simulink model "sphere_portal_mech"  (R2017a)
settings: Solver=FixedStepAuto  StartTime=0.0  StopTime=100  FixedStep=0.001  RelTol=1e-2  EnableMultiTasking=on
undefined symbols (not defined in the file): m, rad, s
libraries: mblibv1 x42, simulink x3, instrumentlib x1
settings Model: SimulationMode=accelerator  Creator=ivanp7  LastModifiedBy=ivanp7
settings OptimizationCC: LifeSpan=inf
settings DebuggingCC: AlgebraicLoopMsg=none  SFUnexpectedBacktrackingDiag=warning  SFNoUnconditionalDefaultTransitionDiag=warning  SFExecutionAtInitializationDiag=none
settings GRTTargetCC: TargetLangStandard=C89/C90 (ANSI)  GeneratePreprocessorConditionals=Disable all
settings ConfigComp: CovMetricSettings=dw  CovHtmlReporting=on  CovSaveCumulativeToWorkspaceVar=on  CovSaveSingleToWorkspaceVar=on  CovExternalEMLEnable=off
settings SimMechanicsCC: LastVizWinPosition=[1141 536 560 420]  CamPosition=[4.37083;-0.373326;26.621;]  CamTarget=[4.37083;-0.373326;0;]  CamUpVector=[0;1;0;]  CamHeight=73.1719  VisBackgroundColor=[0.9;0.9;0.95;]  DefaultBodyColor=[1;0;0;]

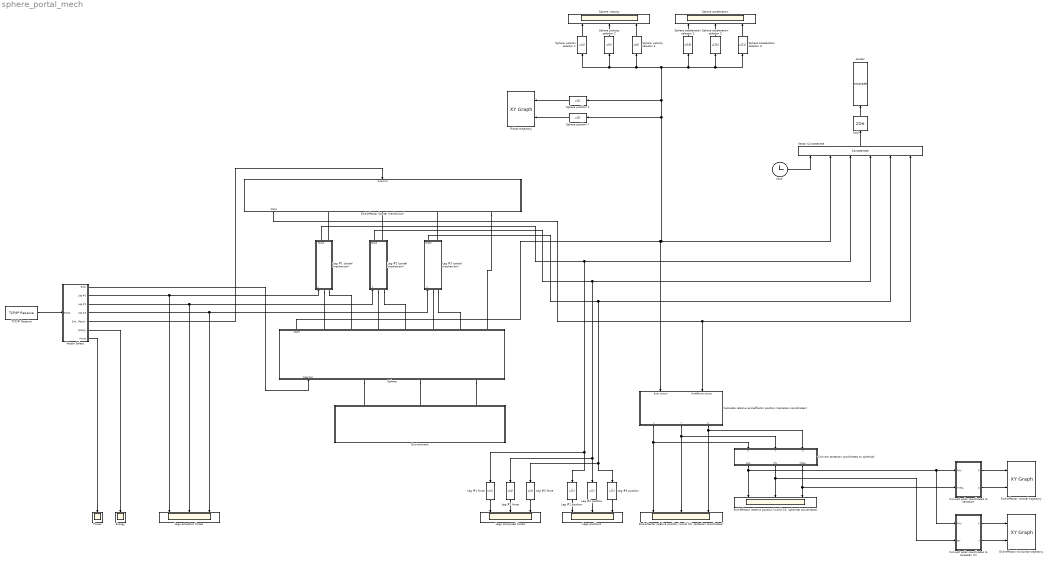
== system sphere_portal_mech ==
  Calculate relative end-effector position (cartesian coordinates) : Subsystem
  Convert cartesian coordinates to spherical : Subsystem
  Convert polar coordinates to cartesian : Subsystem
  Convert polar coordinates to cartesian (2) : Subsystem
  End-effector (portal mechanism) : Subsystem  mask{endeffector_radius=0.2, endeffector_mass=10, endeffector_inertia_coef=2/5}
      mask prompts: endeffector_radius "End-effector radius, m"; endeffector_mass "End-effector mass, kg"; endeffector_inertia_coef "End-effector inertia coefficient"
      mask init:
      | endeffector = endeffector_radius * ...
      |     [[-1; 0; 0], ...
      |      [0; -1; 0], ...
      |      [0; 0; -1], ...
      |      [1; 0; 0], ...
      |      [0; 1; 0], ...
      |      [0; 0; 1]];
  End-effector horizontal trajectory : simulink/Sinks/XY Graph  xmin=-1  xmax=1  ymin=-1  ymax=1  st=-1
  "End-effector relative position (world CS, cartesian coordinates)" : Scope  NumInputPorts=3
  "End-effector relative position (world CS, spherical coordinates)" : Scope  NumInputPorts=3
  End-effector vertical trajectory : simulink/Sinks/XY Graph  xmin=0  xmax=1  ymin=-1  ymax=1  st=-1
  Energy : Scope
  Environment : Subsystem  mask{sphere_radius=1, initial_velocity_x=0, initial_velocity_y=0}
      mask prompts: sphere_radius "Sphere radius, m"; initial_velocity_x "Initial velocity (x-axis), m/s"; initial_velocity_y "Initial velocity (y-axis), m/s"
  Leg #1 force : Fcn  Expr=u(4)
  Leg #1 position : Fcn  Expr=u(1)
  Leg #1 (portal mechanism) : Subsystem  mask{leg_mass=0.1, sphere_radius=1, p_axis=[1 0 0], transient_time=0.001}
      mask prompts: leg_mass "Leg mass, kg"; sphere_radius "Sphere radius, m"; p_axis "Prismatic joint axis"; transient_time "Derivative transient time"
      mask init:
      | p_axis = p_axis / sqrt(sum(p_axis.^2));
      | 
      | v = rand(1, 3);
      | inplane_axis1 = cross(v, p_axis);
      | inplane_axis1 = inplane_axis1 / sqrt(sum(inplane_axis1.^2));
      | inplane_axis2 = cross(inplane_axis1, p_axis);
  Leg #2 force : Fcn  Expr=u(4)
  Leg #2 position : Fcn  Expr=u(1)
  Leg #2 (portal mechanism) : Subsystem  mask{leg_mass=0.1, sphere_radius=1, p_axis=[0 1 0], transient_time=0.001}
      mask prompts: leg_mass "Leg mass, kg"; sphere_radius "Sphere radius, m"; p_axis "Prismatic joint axis"; transient_time "Derivative transient time"
      mask init:
      | p_axis = p_axis / sqrt(sum(p_axis.^2));
      | 
      | v = rand(1, 3);
      | inplane_axis1 = cross(v, p_axis);
      | inplane_axis1 = inplane_axis1 / sqrt(sum(inplane_axis1.^2));
      | inplane_axis2 = cross(inplane_axis1, p_axis);
  Leg #3 force : Fcn  Expr=u(4)
  Leg #3 position : Fcn  Expr=u(1)
  Leg #3 (portal mechanism) : Subsystem  mask{leg_mass=0.1, sphere_radius=1, p_axis=[0 0 1], transient_time=0.001}
      mask prompts: leg_mass "Leg mass, kg"; sphere_radius "Sphere radius, m"; p_axis "Prismatic joint axis"; transient_time "Derivative transient time"
      mask init:
      | p_axis = p_axis / sqrt(sum(p_axis.^2));
      | 
      | v = rand(1, 3);
      | inplane_axis1 = cross(v, p_axis);
      | inplane_axis1 = inplane_axis1 / sqrt(sum(inplane_axis1.^2));
      | inplane_axis2 = cross(inplane_axis1, p_axis);
  Legs actuators forces : Scope  NumInputPorts=3
  Legs computed forces : Scope  NumInputPorts=3
  Legs positions : Scope  NumInputPorts=3
  Power : Scope
  Robot trajectory : simulink/Sinks/XY Graph  xmin=-100  xmax=100  ymin=-100  ymax=100  st=-1
  Sphere : Subsystem  mask{sphere_radius=1, sphere_mass=1, sphere_inertia_coef=2/3}
      mask prompts: sphere_radius "Sphere radius, m"; sphere_mass "Sphere mass, kg"; sphere_inertia_coef "Sphere inertia coefficient, m"
      mask init:
      | cube_side_center = sphere_radius / sqrt(3) * ...
      |     [[-1; 0; 0], ...
      |      [0; -1; 0], ...
      |      [0; 0; -1], ...
      |      [1; 0; 0], ...
      |      [0; 1; 0], ...
      |      [0; 0; 1]];
  Sphere acceleration selector 1 : Fcn  Expr=u(19)
  Sphere acceleration selector 2 : Fcn  Expr=u(20)
  Sphere acceleration selector 3 : Fcn  Expr=u(21)
  Sphere velocity selector 1 : Fcn  Expr=u(4)
  Sphere velocity selector 2 : Fcn  Expr=u(5)
  Sphere velocity selector 3 : Fcn  Expr=u(6)
  Sphere acceleration : Scope  NumInputPorts=3
  Sphere position X : Fcn  Expr=u(1)
  Sphere position Y : Fcn  Expr=u(2)
  Sphere velocity : Scope  NumInputPorts=3
  TCP/IP Receive : instrumentlib/TCP//IP Receive  Priority=1  Host=localhost  Port=61111  DataSize="[1  17]"  EnableBlockingMode=on  Timeout=1  SampleTime=0.001  DataType=double  ByteOrder=LittleEndian
      settings: SourceProductName=Instrument Control Toolbox
  Vector Concatenate : Concatenate  NumInputs=6
  Vector Select : Subsystem
  clock : Clock
      settings: Decimation=1000
  hold : ZeroOrderHold  SampleTime=-1
  sender : M-S-Function  Priority=2  DialogController=instrumentcreatedialog  FunctionName=stcpipsb  Parameters=Host, Port, EnableBlockingMode, Timeout, ByteOrder  DisplayMFileStacktrace=off  mask(TCP/IP Send){Host=localhost, Port=61112, EnableBlockingMode=on, Timeout=1, ByteOrder=LittleEndian}
      mask prompts: Port "Remote Port:"; EnableBlockingMode "Enable blocking mode"; ByteOrder "Byte order:"
      mask help: Send data over TCP/IP network to a specified remote machine.
      mask init:
      | [str port] = instrumentslgate('privateslgetdisplaystring', EnableBlockingMode);
      mask Help: eval('helpview(fullfile(docroot, ''toolbox'', ''instrument'', ''instrument.map''), ''ICT_tcpipsend_Block'')');
      mask TypeOptions ByteOrder: BigEndian | LittleEndian
      mask Display:
      | disp(str);
      | port_label('input',port(1).id,port(1).label);
  wires:
  Leg #1 (portal mechanism)/1(State) -> Leg #1 force/1, Leg #1 position/1, Vector Concatenate/3
  Leg #2 (portal mechanism)/1(State) -> Leg #2 force/1, Leg #2 position/1, Vector Concatenate/4
  Leg #3 (portal mechanism)/1(State) -> Leg #3 force/1, Leg #3 position/1, Vector Concatenate/5
  End-effector (portal mechanism)/1(State) -> Calculate relative end-effector position (cartesian coordinates)/2(Endeffector sensor), Vector Concatenate/6
  Leg #1 position/1 -> Legs positions/1
  Leg #2 position/1 -> Legs positions/2
  Leg #3 position/1 -> Legs positions/3
  Vector Select/4(Leg #3) -> Leg #3 (portal mechanism)/1(Reaction), Legs actuators forces/3
  Vector Select/2(Leg #1) -> Leg #1 (portal mechanism)/1(Reaction), Legs actuators forces/1
  Vector Select/3(Leg #2) -> Leg #2 (portal mechanism)/1(Reaction), Legs actuators forces/2
  Vector Select/5(End effector) -> End-effector (portal mechanism)/1(Reaction)
  Vector Select/1(Body) -> Sphere/1(Reaction)
  Sphere velocity selector 3/1 -> Sphere velocity/3
  Sphere acceleration selector 1/1 -> Sphere acceleration/1
  Sphere acceleration selector 2/1 -> Sphere acceleration/2
  Sphere acceleration selector 3/1 -> Sphere acceleration/3
  Sphere velocity selector 2/1 -> Sphere velocity/2
  Sphere velocity selector 1/1 -> Sphere velocity/1
  Vector Select/6(Energy) -> Energy/1
  Sphere/1(State) -> Vector Concatenate/2, Sphere position X/1, Sphere velocity selector 2/1, Sphere velocity selector 1/1, Sphere velocity selector 3/1, Sphere acceleration selector 1/1, Sphere acceleration selector 2/1, Sphere acceleration selector 3/1, Sphere position Y/1, Calculate relative end-effector position (cartesian coordinates)/1(Body sensor)
  Calculate relative end-effector position (cartesian coordinates)/1(X) -> "End-effector relative position (world CS, cartesian coordinates)"/1, Convert cartesian coordinates to spherical/1(X)
  Calculate relative end-effector position (cartesian coordinates)/2(Y) -> "End-effector relative position (world CS, cartesian coordinates)"/2, Convert cartesian coordinates to spherical/2(Y)
  Calculate relative end-effector position (cartesian coordinates)/3(Z) -> "End-effector relative position (world CS, cartesian coordinates)"/3, Convert cartesian coordinates to spherical/3(Z)
  Convert cartesian coordinates to spherical/1(Rho) -> Convert polar coordinates to cartesian (2)/1(Rho), Convert polar coordinates to cartesian/1(Rho), "End-effector relative position (world CS, spherical coordinates)"/1
  Convert cartesian coordinates to spherical/2(Phi) -> Convert polar coordinates to cartesian (2)/2(Phi), "End-effector relative position (world CS, spherical coordinates)"/2
  Convert cartesian coordinates to spherical/3(Theta) -> Convert polar coordinates to cartesian/2(Theta), "End-effector relative position (world CS, spherical coordinates)"/3
  TCP/IP Receive/1 -> Vector Select/1(Robot)
  hold/1 -> sender/1
  Vector Concatenate/1 -> hold/1
  clock/1 -> Vector Concatenate/1
  Leg #2 force/1 -> Legs computed forces/2
  Leg #1 force/1 -> Legs computed forces/1
  Leg #3 force/1 -> Legs computed forces/3
  Vector Select/7(Power) -> Power/1
  Sphere position X/1 -> Robot trajectory/1
  Sphere position Y/1 -> Robot trajectory/2
  Convert polar coordinates to cartesian/1(R) -> End-effector vertical trajectory/1
  Convert polar coordinates to cartesian/2(Z) -> End-effector vertical trajectory/2
  Convert polar coordinates to cartesian (2)/2(Y) -> End-effector horizontal trajectory/2
  Convert polar coordinates to cartesian (2)/1(X) -> End-effector horizontal trajectory/1
  connections:
  Leg #1 (portal mechanism)/LConn1 -- Sphere/RConn1
  Leg #1 (portal mechanism)/LConn2 -- Sphere/RConn2
  Sphere/LConn1 -- Environment/LConn1
  Sphere/LConn2 -- Environment/LConn2
  Sphere/LConn3 -- Environment/LConn3
  Leg #1 (portal mechanism)/RConn1 -- End-effector (portal mechanism)/RConn1
  End-effector (portal mechanism)/RConn4 -- Sphere/RConn7
  Leg #2 (portal mechanism)/RConn1 -- End-effector (portal mechanism)/RConn2
  Leg #3 (portal mechanism)/RConn1 -- End-effector (portal mechanism)/RConn3
  Leg #2 (portal mechanism)/LConn1 -- Sphere/RConn3
  Leg #2 (portal mechanism)/LConn2 -- Sphere/RConn4
  Leg #3 (portal mechanism)/LConn1 -- Sphere/RConn5
  Leg #3 (portal mechanism)/LConn2 -- Sphere/RConn6

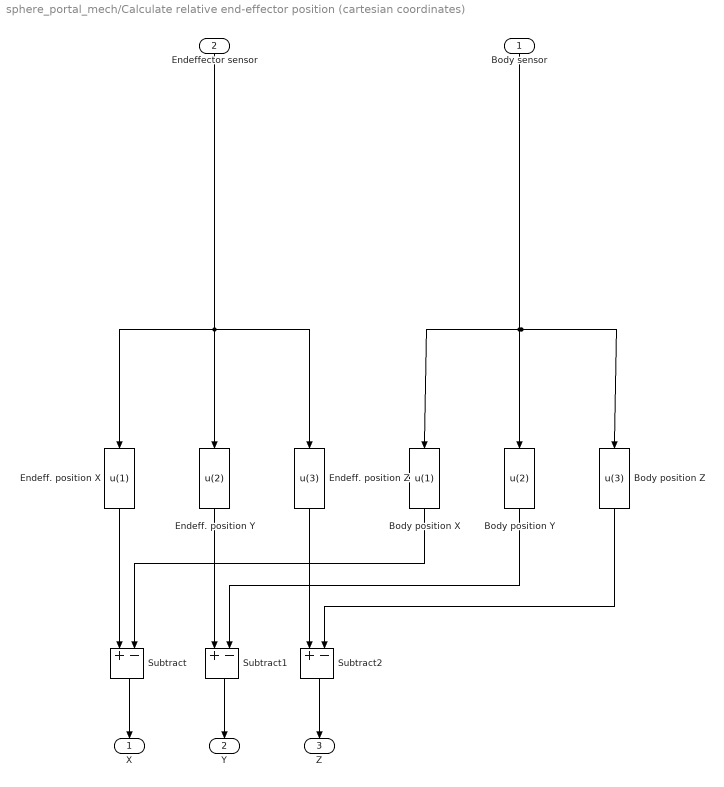
== system sphere_portal_mech/Calculate relative end-effector position (cartesian coordinates) ==
  Body sensor : Inport
  Endeffector sensor : Inport  Port=2
  Body position X : Fcn  Expr=u(1)
  Body position Y : Fcn  Expr=u(2)
  Body position Z : Fcn  Expr=u(3)
  Endeff. position X : Fcn  Expr=u(1)
  Endeff. position Y : Fcn  Expr=u(2)
  Endeff. position Z : Fcn  Expr=u(3)
  Subtract : Sum  Inputs=+-
  Subtract1 : Sum  Inputs=+-
  Subtract2 : Sum  Inputs=+-
  X : Outport
  Y : Outport  Port=2
  Z : Outport  Port=3
  wires:
  Body position X/1 -> Subtract/2
  Body position Z/1 -> Subtract2/2
  Subtract/1 -> X/1
  Subtract1/1 -> Y/1
  Endeff. position X/1 -> Subtract/1
  Endeff. position Y/1 -> Subtract1/1
  Endeff. position Z/1 -> Subtract2/1
  Subtract2/1 -> Z/1
  Body sensor/1 -> Body position Z/1, Body position Y/1, Body position X/1
  Body position Y/1 -> Subtract1/2
  Endeffector sensor/1 -> Endeff. position Z/1, Endeff. position X/1, Endeff. position Y/1

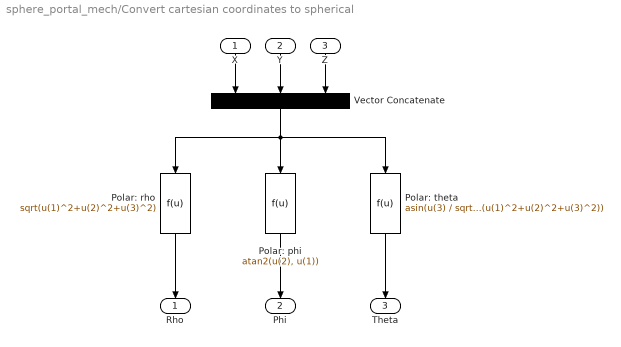
== system sphere_portal_mech/Convert cartesian coordinates to spherical ==
  X : Inport
  Y : Inport  Port=2
  Z : Inport  Port=3
  Polar: phi : Fcn  Expr=atan2(u(2), u(1))
  Polar: rho : Fcn  Expr=sqrt(u(1)^2+u(2)^2+u(3)^2)
  Polar: theta : Fcn  Expr=asin(u(3) / sqrt(u(1)^2+u(2)^2+u(3)^2))
  Vector Concatenate : Concatenate  NumInputs=3
  Rho : Outport
  Phi : Outport  Port=2
  Theta : Outport  Port=3
  wires:
  Polar: rho/1 -> Rho/1
  Polar: phi/1 -> Phi/1
  Polar: theta/1 -> Theta/1
  Y/1 -> Vector Concatenate/2
  Z/1 -> Vector Concatenate/3
  X/1 -> Vector Concatenate/1
  Vector Concatenate/1 -> Polar: theta/1, Polar: rho/1, Polar: phi/1

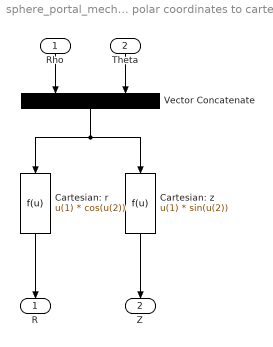
== system sphere_portal_mech/Convert polar coordinates to cartesian ==
  Rho : Inport
  Theta : Inport  Port=2
  Cartesian: r : Fcn  Expr=u(1) * cos(u(2))
  Cartesian: z : Fcn  Expr=u(1) * sin(u(2))
  Vector Concatenate : Concatenate
  R : Outport
  Z : Outport  Port=2
  wires:
  Cartesian: r/1 -> R/1
  Cartesian: z/1 -> Z/1
  Theta/1 -> Vector Concatenate/2
  Rho/1 -> Vector Concatenate/1
  Vector Concatenate/1 -> Cartesian: z/1, Cartesian: r/1

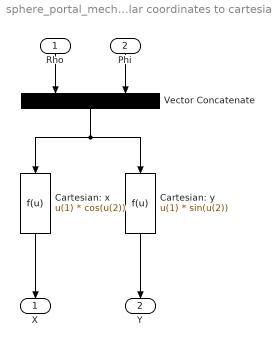
== system sphere_portal_mech/Convert polar coordinates to cartesian (2) ==
  Rho : Inport
  Phi : Inport  Port=2
  Cartesian: x : Fcn  Expr=u(1) * cos(u(2))
  Cartesian: y : Fcn  Expr=u(1) * sin(u(2))
  Vector Concatenate : Concatenate
  X : Outport
  Y : Outport  Port=2
  wires:
  Cartesian: x/1 -> X/1
  Cartesian: y/1 -> Y/1
  Phi/1 -> Vector Concatenate/2
  Rho/1 -> Vector Concatenate/1
  Vector Concatenate/1 -> Cartesian: y/1, Cartesian: x/1

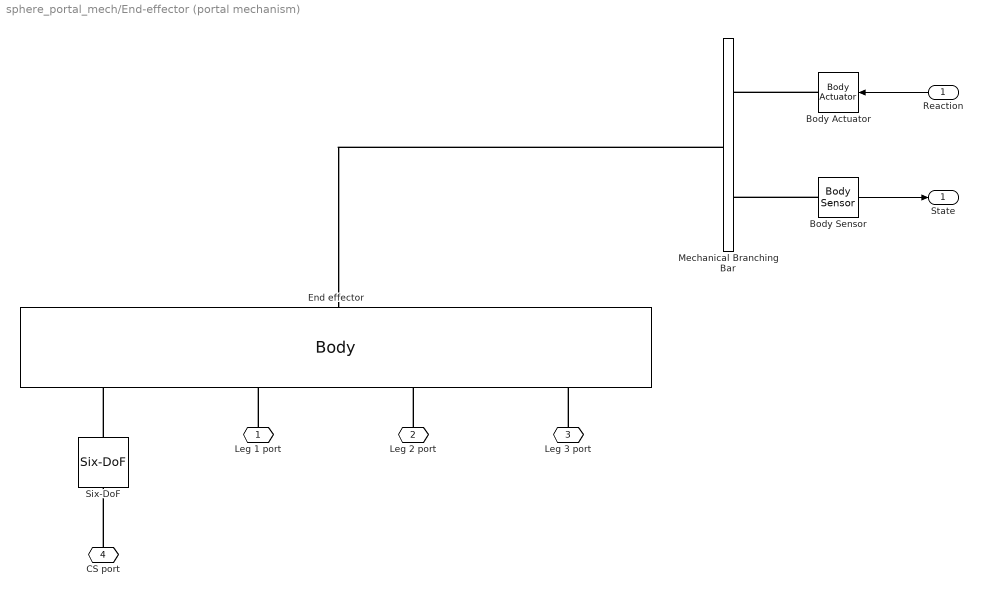
== system sphere_portal_mech/End-effector (portal mechanism) ==
  Reaction : Inport  OutDataTypeStr=double
  Body Actuator : mblibv1/Sensors &  Actuators/Body Actuator  UpdateFromCAD=off  PhysicalDomain=Mechanical  PortType=blob  ActuationStyle=Force  AngleUnits=deg  ArcVelocityUnits=deg/s  ArcAccelerationUnits=deg/s^2  CoordPositionUnits=m  VelocityUnits=m/s  AccelerationUnits=m/s^2  ForceUnits=N  TorqueUnits=N*m  ActiveIO=on  Width=6  DialogClass=MechanicalActuatorBlock  ReferenceFrame=Absolute (World)  Angle=off  CoordPosition=on  Force=on  Torque=on
      settings: SourceProductName=Simscape Multibody  SourceProductBaseCode=MS
  Body Sensor : mblibv1/Sensors &  Actuators/Body Sensor  UpdateFromCAD=off  PhysicalDomain=Mechanical  PortType=blob  Muxed=on  Pose=on  Angle=on  AngleUnits=deg  ArcVelocity=on  ArcVelocityUnits=rad/s  ArcAcceleration=on  ArcAccelerationUnits=rad/s^2  CoordPosition=on  CoordPositionUnits=m  Velocity=on  VelocityUnits=m/s  Acceleration=on  AccelerationUnits=m/s^2  Quaternion=on  QuaternionDT=off  QuaternionDDT=off  QuaternionUnits=off  OutputVector=[1]  ActiveIO=on  Width=24  DialogClass=MechanicalSensorBlock  ReferenceFrame=Absolute (World)
      settings: SourceProductName=Simscape Multibody  SourceProductBaseCode=MS
  End effector : mblibv1/Bodies/Body  LConnTagsString=CS7  RConnTagsString=CG|CS8|CS9|CS10  UpdateFromCAD=off  DialogClass=MechanicalBodyBlock  Mass=endeffector_mass  MassUnits=kg  InertiaUnits=kg*m^2  Inertia=endeffector_inertia_coef*endeffector_mass*endeffector_radius^2*eye(3)  Shape=Cylinder  ShapeDims=[1 1]  ShapeUnits=m  ShapeUse=false  Density=1  DensityUnits=kg/m^3  DensityUse=false  GraphicsMode=CONVHULL  BodyColorSelMode=MACHINE_DEFAULT  BodyColor=[1 0 0]  AttachedToCS=CG  CG=Right$CG$[0;0;0]$Adjoining$Adjoining$m$[0 0 0]$Euler X-Y-Z$deg$Adjoining$true$none  WorkingFrames=Right$CS1$endeffector(:, 1)$CG$CG$m$[0 0 0]$Euler X-Y-Z$deg$CG$false$none#Right$CS2$endeffector(:, 2)$CG$CG$m$[0 0 0]$Euler X-Y-Z$deg$CG$false$none#Right$CS3$endeffector(:, 3)$CG$CG$m$[0 0 0]$Euler X-Y-Z$deg$CG$false$none#Right$CS4$endeffector(:, 4)$CG$CG$m$[0 0 0]$Euler X-Y-Z$deg$CG$false$none#Right$CS5$endeffector(:, 5)$CG$CG$m$[0 0 0]$Euler X-Y-Z$deg$CG$false$none#Right$CS6$endeffector(:, 6)$CG$CG$m$[0 0 0]$Euler X-Y-Z$deg$CG$false$none#Left$CS7$[0;0;0]$CG$CG$m$[0 0 0]$Euler X-Y-Z$deg$CG$true$none#Right$CS8$[0;0;0]$CG$CG$m$[0 0 0]$Euler X-Y-Z$deg$CG$true$none#Right$CS9$[0;0;0]$CG$CG$m$[0 0 0]$Euler X-Y-Z$deg$CG$true$none#Right$CS10$[0;0;0]$CG$CG$m$[0 0 0]$Euler X-Y-Z$deg$CG$true$none  CGPos=[0;0;0]  CGRot=[0 0 0]  CS0Pos=[]  CS0Rot=[]  CS1Pos=endeffector(:, 1)  CS1Rot=[0 0 0]  CS2Pos=endeffector(:, 2)  CS2Rot=[0 0 0]  CS3Pos=endeffector(:, 3)  CS3Rot=[0 0 0]  CS4Pos=endeffector(:, 4)  CS4Rot=[0 0 0]  CS5Pos=endeffector(:, 5)  CS5Rot=[0 0 0]  CS6Pos=endeffector(:, 6)  CS6Rot=[0 0 0]  CS7Pos=[0;0;0]  CS7Rot=[0 0 0]  CS8Pos=[0;0;0]  CS8Rot=[0 0 0]  CS9Pos=[0;0;0]  CS9Rot=[0 0 0]  CS10Pos=[0;0;0]  CS10Rot=[0 0 0]  CS11Pos=[]  CS11Rot=[]  CS12Pos=[]  CS12Rot=[]  CS13Pos=[]  CS13Rot=[]  CS14Pos=[]  CS14Rot=[]  CS15Pos=[]  CS15Rot=[]  CS16Pos=[]  CS16Rot=[]  CS17Pos=[]  CS17Rot=[]  CS18Pos=[]  CS18Rot=[]  CS19Pos=[]  CS19Rot=[]  CS20Pos=[]  CS20Rot=[]
      settings: SourceProductName=Simscape Multibody  SourceProductBaseCode=MS
  Mechanical Branching Bar : mblibv1/Utilities/Mechanical Branching Bar  LConnTagsString=_newl0  RConnTagsString=SA0|SA1  UpdateFromCAD=off  DialogClass=MechanicalBranchingBarBlock  NumSAPorts=2
      settings: SourceProductName=Simscape Multibody  SourceProductBaseCode=MS
  Six-DoF : mblibv1/Joints/Six-DoF  LConnTagsString=__newl0  RConnTagsString=__newr0  UpdateFromCAD=off  NumSAPorts=0  CutJoint=off  MarkAsCut=off  Primitives=prismatic_prismatic  PrimitiveProps=P1$WORLD$[1 0 0]$prismatic#P2$WORLD$[0 1 0]$prismatic#P3$WORLD$[0 0 1]$prismatic#S$WORLD$[0 0 0]$spherical  DialogClass=JointBlock  P1Axis=[1 0 0]  P2Axis=[0 1 0]  P3Axis=[0 0 1]  SAxis=[0 0 0]
      settings: SourceProductName=Simscape Multibody  SourceProductBaseCode=MS
  Leg 1 port : PMIOPort  Port=1  Side=Right
  Leg 2 port : PMIOPort  Port=2  Side=Right
  Leg 3 port : PMIOPort  Port=3  Side=Right
  CS port : PMIOPort  Port=4  Side=Right
  State : Outport  OutDataTypeStr=double
  wires:
  Reaction/1 -> Body Actuator/1
  Body Sensor/1 -> State/1
  connections:
  Mechanical Branching Bar/LConn1 -- End effector/LConn1
  Leg 2 port/RConn1 -- End effector/RConn3
  Leg 3 port/RConn1 -- End effector/RConn4
  Leg 1 port/RConn1 -- End effector/RConn2
  Body Actuator/RConn1 -- Mechanical Branching Bar/RConn1
  Six-DoF/RConn1 -- End effector/RConn1
  Body Sensor/LConn1 -- Mechanical Branching Bar/RConn2
  CS port/RConn1 -- Six-DoF/LConn1

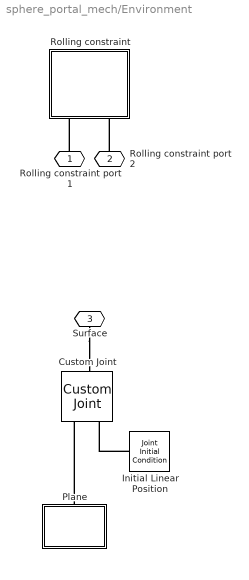
== system sphere_portal_mech/Environment ==
  Custom Joint : mblibv1/Joints/Custom Joint  LConnTagsString=__newl0|SA1  RConnTagsString=__newr0  UpdateFromCAD=off  NumSAPorts=1  CutJoint=off  MarkAsCut=off  Primitives=prismatic_prismatic_spherical  PrimitiveProps=P1$World$[1 0 0]$prismatic#P2$World$[0 1 0]$prismatic#S$World$[0 0 0]$spherical  DialogClass=JointBlock  R1Axis=[]  R2Axis=[]  R3Axis=[]  P1Axis=[1 0 0]  P2Axis=[0 1 0]  P3Axis=[]  SAxis=[0 0 0]
      settings: SourceProductName=Simscape Multibody  SourceProductBaseCode=MS
  Initial Linear Position : mblibv1/Sensors &  Actuators/Joint Initial Condition  UpdateFromCAD=off  LeftPortType=blob  RightPortType=blob  PhysicalDomain=Mechanical  DialogClass=InitialConditionBlock  InitialConditions=P1$true$0$m$rad$initial_velocity_x$m/s$rad/s#P2$true$0$m$rad$initial_velocity_y$m/s$rad/s#P3$false$0$m$rad$0$m/s$rad/s#R1$false$0$m$rad$0$m/s$rad/s#R2$false$0$m$rad$0$m/s$rad/s#R3$false$0$m$rad$0$m/s$rad/s#S$false$0$m$rad$0$m/s$rad/s  P1PIC=0  P1VIC=initial_velocity_x  P2PIC=0  P2VIC=initial_velocity_y  P3PIC=0  P3VIC=0  R1PIC=0  R1VIC=0  R2PIC=0  R2VIC=0  R3PIC=0  R3VIC=0  SPIC=0  SVIC=0
      settings: SourceProductName=Simscape Multibody  SourceProductBaseCode=MS
  Plane : Subsystem  mask{width=5}
      mask prompts: width "Square width"
  Rolling constraint : Subsystem
  Rolling constraint port 1 : PMIOPort  Port=1  Side=Left
  Rolling constraint port 2 : PMIOPort  Port=2  Side=Left
  Surface : PMIOPort  Port=3  Side=Left
  connections:
  Surface/RConn1 -- Custom Joint/RConn1
  Plane/LConn1 -- Custom Joint/LConn1
  Initial Linear Position/RConn1 -- Custom Joint/LConn2
  Rolling constraint port 2/RConn1 -- Rolling constraint/LConn2
  Rolling constraint port 1/RConn1 -- Rolling constraint/LConn1

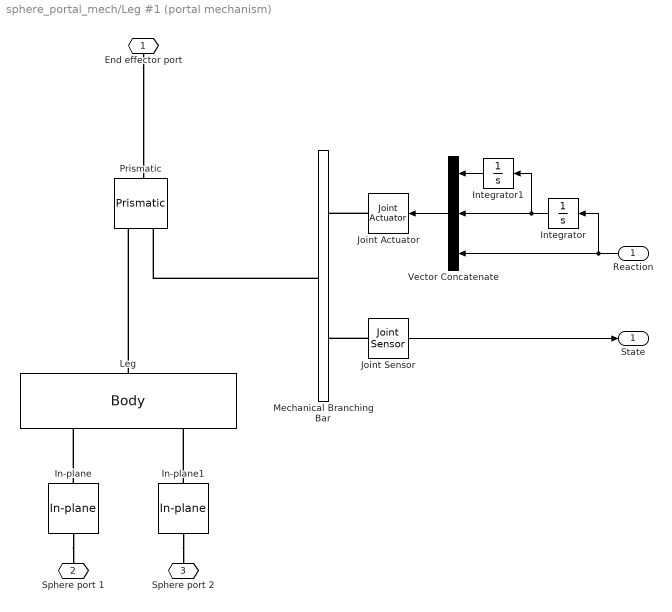
== system sphere_portal_mech/Leg #1 (portal mechanism) ==
  Reaction : Inport
  In-plane : mblibv1/Joints/In-plane  LConnTagsString=__newl0  RConnTagsString=__newr0  UpdateFromCAD=off  NumSAPorts=0  CutJoint=off  MarkAsCut=off  Primitives=prismatic  PrimitiveProps=P1$Base$inplane_axis1$prismatic#P2$Base$inplane_axis2$prismatic  DialogClass=JointBlock  P1Axis=inplane_axis1  P2Axis=inplane_axis2
      settings: SourceProductName=Simscape Multibody  SourceProductBaseCode=MS
  In-plane1 : mblibv1/Joints/In-plane  LConnTagsString=__newl0  RConnTagsString=__newr0  UpdateFromCAD=off  NumSAPorts=0  CutJoint=off  MarkAsCut=off  Primitives=prismatic  PrimitiveProps=P1$Base$inplane_axis1$prismatic#P2$Base$inplane_axis2$prismatic  DialogClass=JointBlock  P1Axis=inplane_axis1  P2Axis=inplane_axis2
      settings: SourceProductName=Simscape Multibody  SourceProductBaseCode=MS
  Integrator : Integrator
  Integrator1 : Integrator
  Joint Actuator : mblibv1/Sensors &  Actuators/Joint Actuator  UpdateFromCAD=off  PhysicalDomain=Mechanical  PortType=blob  ActuationStyle=Motion  AngleUnits=deg  ArcVelocityUnits=deg/s  ArcAccelerationUnits=deg/s^2  CoordPositionUnits=m  VelocityUnits=m/s  AccelerationUnits=m/s^2  ForceUnits=N  TorqueUnits=N*m  ActiveIO=on  Width=3  DialogClass=MechanicalActuatorBlock  Primitive=P1  ReferenceFrame=Absolute (World)
      settings: SourceProductName=Simscape Multibody  SourceProductBaseCode=MS
  Joint Sensor : mblibv1/Sensors &  Actuators/Joint Sensor  UpdateFromCAD=off  PhysicalDomain=Mechanical  PortType=blob  Muxed=on  Pose=off  Angle=on  AngleUnits=deg  ArcVelocity=off  ArcVelocityUnits=deg/s  ArcAcceleration=off  ArcAccelerationUnits=deg/s^2  CoordPosition=on  CoordPositionUnits=m  Velocity=on  VelocityUnits=m/s  Acceleration=on  AccelerationUnits=m/s^2  Quaternion=on  QuaternionDT=off  QuaternionDDT=off  QuaternionUnits=off  OutputVector=[1]  ActiveIO=on  Width=10  DialogClass=MechanicalSensorBlock  Primitive=P1  Force=on  ForceUnits=N  Torque=off  TorqueUnits=N*m  ReferenceFrame=Absolute (World)  ReactionSensedSide=Base  ReactionReferenceFrame=Local (Body CS)  ReactionForce=on  ReactionForceUnits=N  ReactionMoment=on  ReactionMomentUnits=N*m
      settings: SourceProductName=Simscape Multibody  SourceProductBaseCode=MS
  Leg : mblibv1/Bodies/Body  LConnTagsString=CG  RConnTagsString=CS1|CS2  UpdateFromCAD=off  DialogClass=MechanicalBodyBlock  Mass=leg_mass  MassUnits=kg  InertiaUnits=kg*m^2  Inertia=zeros(3)  Shape=Cylinder  ShapeDims=[1 1]  ShapeUnits=m  ShapeUse=false  Density=1  DensityUnits=kg/m^3  DensityUse=false  GraphicsMode=CONVHULL  BodyColorSelMode=COLORPALETTE  BodyColor=[0 1 0]  AttachedToCS=CG  CG=Left$CG$[0 0 0]$Adjoining$Adjoining$m$[0 0 0]$Euler X-Y-Z$deg$Adjoining$true$none  WorkingFrames=Right$CS1$[0 0 0]$Adjoining$Adjoining$m$[0 0 0]$Euler X-Y-Z$deg$Adjoining$true$none#Right$CS2$[0 0 0]$Adjoining$Adjoining$m$[0 0 0]$Euler X-Y-Z$deg$Adjoining$true$none  CGPos=[0 0 0]  CGRot=[0 0 0]  CS0Pos=[]  CS0Rot=[]  CS1Pos=[0 0 0]  CS1Rot=[0 0 0]  CS2Pos=[0 0 0]  CS2Rot=[0 0 0]  CS3Pos=[]  CS3Rot=[]  CS4Pos=[]  CS4Rot=[]  CS5Pos=[]  CS5Rot=[]  CS6Pos=[]  CS6Rot=[]  CS7Pos=[]  CS7Rot=[]  CS8Pos=[]  CS8Rot=[]  CS9Pos=[]  CS9Rot=[]  CS10Pos=[]  CS10Rot=[]  CS11Pos=[]  CS11Rot=[]  CS12Pos=[]  CS12Rot=[]  CS13Pos=[]  CS13Rot=[]  CS14Pos=[]  CS14Rot=[]  CS15Pos=[]  CS15Rot=[]  CS16Pos=[]  CS16Rot=[]  CS17Pos=[]  CS17Rot=[]  CS18Pos=[]  CS18Rot=[]  CS19Pos=[]  CS19Rot=[]  CS20Pos=[]  CS20Rot=[]
      settings: SourceProductName=Simscape Multibody  SourceProductBaseCode=MS
  Mechanical Branching Bar : mblibv1/Utilities/Mechanical Branching Bar  LConnTagsString=_newl0  RConnTagsString=SA0|SA1  UpdateFromCAD=off  DialogClass=MechanicalBranchingBarBlock  NumSAPorts=2
      settings: SourceProductName=Simscape Multibody  SourceProductBaseCode=MS
  Prismatic : mblibv1/Joints/Prismatic  LConnTagsString=__newl0|SA1  RConnTagsString=__newr0  UpdateFromCAD=off  NumSAPorts=1  CutJoint=on  MarkAsCut=off  Primitives=prismatic  PrimitiveProps=P1$Base$p_axis$prismatic  DialogClass=JointBlock  P1Axis=p_axis
      settings: SourceProductName=Simscape Multibody  SourceProductBaseCode=MS
  Vector Concatenate : Concatenate  NumInputs=3
  End effector port : PMIOPort  Port=1  Side=Right
  Sphere port 1 : PMIOPort  Port=2  Side=Left
  Sphere port 2 : PMIOPort  Port=3  Side=Left
  State : Outport
  wires:
  Joint Sensor/1 -> State/1
  Vector Concatenate/1 -> Joint Actuator/1
  Reaction/1 -> Integrator/1, Vector Concatenate/3
  Integrator/1 -> Integrator1/1, Vector Concatenate/2
  Integrator1/1 -> Vector Concatenate/1
  connections:
  End effector port/RConn1 -- Prismatic/RConn1
  In-plane/RConn1 -- Leg/RConn1
  Leg/LConn1 -- Prismatic/LConn1
  In-plane/LConn1 -- Sphere port 1/RConn1
  Joint Actuator/RConn1 -- Mechanical Branching Bar/RConn1
  In-plane1/LConn1 -- Sphere port 2/RConn1
  In-plane1/RConn1 -- Leg/RConn2
  Mechanical Branching Bar/LConn1 -- Prismatic/LConn2
  Joint Sensor/LConn1 -- Mechanical Branching Bar/RConn2

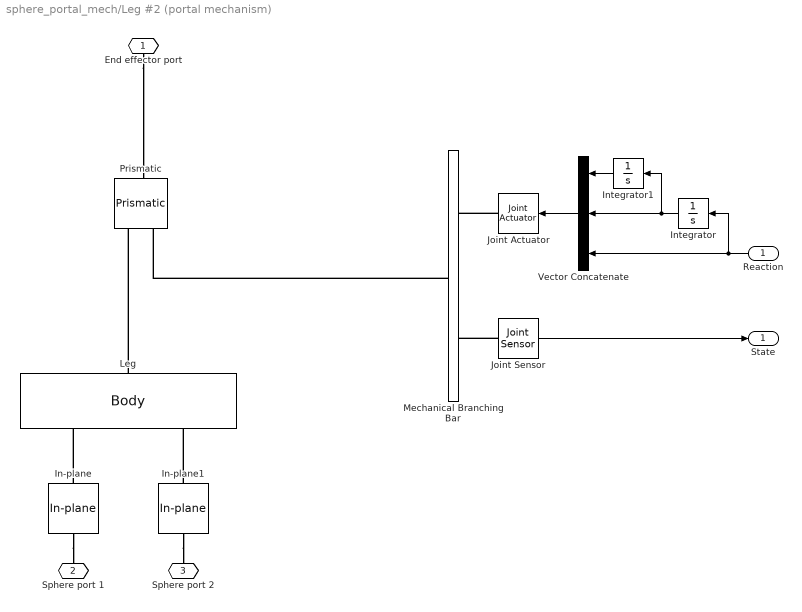
== system sphere_portal_mech/Leg #2 (portal mechanism) ==
  Reaction : Inport
  In-plane : mblibv1/Joints/In-plane  LConnTagsString=__newl0  RConnTagsString=__newr0  UpdateFromCAD=off  NumSAPorts=0  CutJoint=off  MarkAsCut=off  Primitives=prismatic  PrimitiveProps=P1$Base$inplane_axis1$prismatic#P2$Base$inplane_axis2$prismatic  DialogClass=JointBlock  P1Axis=inplane_axis1  P2Axis=inplane_axis2
      settings: SourceProductName=Simscape Multibody  SourceProductBaseCode=MS
  In-plane1 : mblibv1/Joints/In-plane  LConnTagsString=__newl0  RConnTagsString=__newr0  UpdateFromCAD=off  NumSAPorts=0  CutJoint=off  MarkAsCut=off  Primitives=prismatic  PrimitiveProps=P1$Base$inplane_axis1$prismatic#P2$Base$inplane_axis2$prismatic  DialogClass=JointBlock  P1Axis=inplane_axis1  P2Axis=inplane_axis2
      settings: SourceProductName=Simscape Multibody  SourceProductBaseCode=MS
  Integrator : Integrator
  Integrator1 : Integrator
  Joint Actuator : mblibv1/Sensors &  Actuators/Joint Actuator  UpdateFromCAD=off  PhysicalDomain=Mechanical  PortType=blob  ActuationStyle=Motion  AngleUnits=deg  ArcVelocityUnits=deg/s  ArcAccelerationUnits=deg/s^2  CoordPositionUnits=m  VelocityUnits=m/s  AccelerationUnits=m/s^2  ForceUnits=N  TorqueUnits=N*m  ActiveIO=on  Width=3  DialogClass=MechanicalActuatorBlock  Primitive=P1  ReferenceFrame=Absolute (World)
      settings: SourceProductName=Simscape Multibody  SourceProductBaseCode=MS
  Joint Sensor : mblibv1/Sensors &  Actuators/Joint Sensor  UpdateFromCAD=off  PhysicalDomain=Mechanical  PortType=blob  Muxed=on  Pose=off  Angle=on  AngleUnits=deg  ArcVelocity=off  ArcVelocityUnits=deg/s  ArcAcceleration=off  ArcAccelerationUnits=deg/s^2  CoordPosition=on  CoordPositionUnits=m  Velocity=on  VelocityUnits=m/s  Acceleration=on  AccelerationUnits=m/s^2  Quaternion=on  QuaternionDT=off  QuaternionDDT=off  QuaternionUnits=off  OutputVector=[1]  ActiveIO=on  Width=10  DialogClass=MechanicalSensorBlock  Primitive=P1  Force=on  ForceUnits=N  Torque=off  TorqueUnits=N*m  ReferenceFrame=Absolute (World)  ReactionSensedSide=Base  ReactionReferenceFrame=Local (Body CS)  ReactionForce=on  ReactionForceUnits=N  ReactionMoment=on  ReactionMomentUnits=N*m
      settings: SourceProductName=Simscape Multibody  SourceProductBaseCode=MS
  Leg : mblibv1/Bodies/Body  LConnTagsString=CG  RConnTagsString=CS1|CS2  UpdateFromCAD=off  DialogClass=MechanicalBodyBlock  Mass=leg_mass  MassUnits=kg  InertiaUnits=kg*m^2  Inertia=zeros(3)  Shape=Cylinder  ShapeDims=[1 1]  ShapeUnits=m  ShapeUse=false  Density=1  DensityUnits=kg/m^3  DensityUse=false  GraphicsMode=CONVHULL  BodyColorSelMode=COLORPALETTE  BodyColor=[0 1 0]  AttachedToCS=CG  CG=Left$CG$[0 0 0]$Adjoining$Adjoining$m$[0 0 0]$Euler X-Y-Z$deg$Adjoining$true$none  WorkingFrames=Right$CS1$[0 0 0]$Adjoining$Adjoining$m$[0 0 0]$Euler X-Y-Z$deg$Adjoining$true$none#Right$CS2$[0 0 0]$Adjoining$Adjoining$m$[0 0 0]$Euler X-Y-Z$deg$Adjoining$true$none  CGPos=[0 0 0]  CGRot=[0 0 0]  CS0Pos=[]  CS0Rot=[]  CS1Pos=[0 0 0]  CS1Rot=[0 0 0]  CS2Pos=[0 0 0]  CS2Rot=[0 0 0]  CS3Pos=[]  CS3Rot=[]  CS4Pos=[]  CS4Rot=[]  CS5Pos=[]  CS5Rot=[]  CS6Pos=[]  CS6Rot=[]  CS7Pos=[]  CS7Rot=[]  CS8Pos=[]  CS8Rot=[]  CS9Pos=[]  CS9Rot=[]  CS10Pos=[]  CS10Rot=[]  CS11Pos=[]  CS11Rot=[]  CS12Pos=[]  CS12Rot=[]  CS13Pos=[]  CS13Rot=[]  CS14Pos=[]  CS14Rot=[]  CS15Pos=[]  CS15Rot=[]  CS16Pos=[]  CS16Rot=[]  CS17Pos=[]  CS17Rot=[]  CS18Pos=[]  CS18Rot=[]  CS19Pos=[]  CS19Rot=[]  CS20Pos=[]  CS20Rot=[]
      settings: SourceProductName=Simscape Multibody  SourceProductBaseCode=MS
  Mechanical Branching Bar : mblibv1/Utilities/Mechanical Branching Bar  LConnTagsString=_newl0  RConnTagsString=SA0|SA1  UpdateFromCAD=off  DialogClass=MechanicalBranchingBarBlock  NumSAPorts=2
      settings: SourceProductName=Simscape Multibody  SourceProductBaseCode=MS
  Prismatic : mblibv1/Joints/Prismatic  LConnTagsString=__newl0|SA1  RConnTagsString=__newr0  UpdateFromCAD=off  NumSAPorts=1  CutJoint=on  MarkAsCut=off  Primitives=prismatic  PrimitiveProps=P1$Follower$p_axis$prismatic  DialogClass=JointBlock  P1Axis=p_axis
      settings: SourceProductName=Simscape Multibody  SourceProductBaseCode=MS
  Vector Concatenate : Concatenate  NumInputs=3
  End effector port : PMIOPort  Port=1  Side=Right
  Sphere port 1 : PMIOPort  Port=2  Side=Left
  Sphere port 2 : PMIOPort  Port=3  Side=Left
  State : Outport
  wires:
  Joint Sensor/1 -> State/1
  Integrator1/1 -> Vector Concatenate/1
  Integrator/1 -> Integrator1/1, Vector Concatenate/2
  Reaction/1 -> Integrator/1, Vector Concatenate/3
  Vector Concatenate/1 -> Joint Actuator/1
  connections:
  End effector port/RConn1 -- Prismatic/RConn1
  In-plane/RConn1 -- Leg/RConn1
  Leg/LConn1 -- Prismatic/LConn1
  In-plane/LConn1 -- Sphere port 1/RConn1
  In-plane1/LConn1 -- Sphere port 2/RConn1
  In-plane1/RConn1 -- Leg/RConn2
  Mechanical Branching Bar/LConn1 -- Prismatic/LConn2
  Joint Actuator/RConn1 -- Mechanical Branching Bar/RConn1
  Joint Sensor/LConn1 -- Mechanical Branching Bar/RConn2

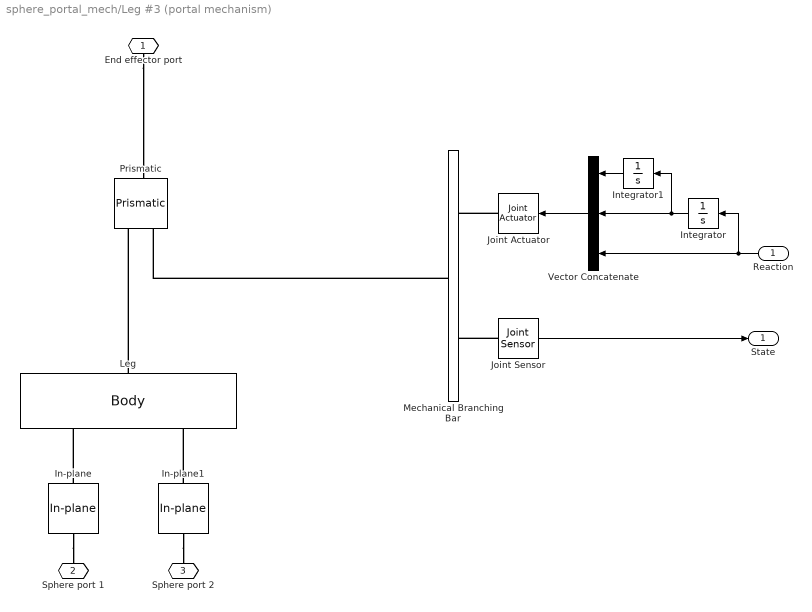
== system sphere_portal_mech/Leg #3 (portal mechanism) ==
  Reaction : Inport
  In-plane : mblibv1/Joints/In-plane  LConnTagsString=__newl0  RConnTagsString=__newr0  UpdateFromCAD=off  NumSAPorts=0  CutJoint=off  MarkAsCut=off  Primitives=prismatic  PrimitiveProps=P1$Base$inplane_axis1$prismatic#P2$Base$inplane_axis2$prismatic  DialogClass=JointBlock  P1Axis=inplane_axis1  P2Axis=inplane_axis2
      settings: SourceProductName=Simscape Multibody  SourceProductBaseCode=MS
  In-plane1 : mblibv1/Joints/In-plane  LConnTagsString=__newl0  RConnTagsString=__newr0  UpdateFromCAD=off  NumSAPorts=0  CutJoint=off  MarkAsCut=off  Primitives=prismatic  PrimitiveProps=P1$Base$inplane_axis1$prismatic#P2$Base$inplane_axis2$prismatic  DialogClass=JointBlock  P1Axis=inplane_axis1  P2Axis=inplane_axis2
      settings: SourceProductName=Simscape Multibody  SourceProductBaseCode=MS
  Integrator : Integrator
  Integrator1 : Integrator
  Joint Actuator : mblibv1/Sensors &  Actuators/Joint Actuator  UpdateFromCAD=off  PhysicalDomain=Mechanical  PortType=blob  ActuationStyle=Motion  AngleUnits=deg  ArcVelocityUnits=deg/s  ArcAccelerationUnits=deg/s^2  CoordPositionUnits=m  VelocityUnits=m/s  AccelerationUnits=m/s^2  ForceUnits=N  TorqueUnits=N*m  ActiveIO=on  Width=3  DialogClass=MechanicalActuatorBlock  Primitive=P1  ReferenceFrame=Absolute (World)
      settings: SourceProductName=Simscape Multibody  SourceProductBaseCode=MS
  Joint Sensor : mblibv1/Sensors &  Actuators/Joint Sensor  UpdateFromCAD=off  PhysicalDomain=Mechanical  PortType=blob  Muxed=on  Pose=off  Angle=on  AngleUnits=deg  ArcVelocity=off  ArcVelocityUnits=deg/s  ArcAcceleration=off  ArcAccelerationUnits=deg/s^2  CoordPosition=on  CoordPositionUnits=m  Velocity=on  VelocityUnits=m/s  Acceleration=on  AccelerationUnits=m/s^2  Quaternion=on  QuaternionDT=off  QuaternionDDT=off  QuaternionUnits=off  OutputVector=[1]  ActiveIO=on  Width=10  DialogClass=MechanicalSensorBlock  Primitive=P1  Force=on  ForceUnits=N  Torque=off  TorqueUnits=N*m  ReferenceFrame=Absolute (World)  ReactionSensedSide=Base  ReactionReferenceFrame=Local (Body CS)  ReactionForce=on  ReactionForceUnits=N  ReactionMoment=on  ReactionMomentUnits=N*m
      settings: SourceProductName=Simscape Multibody  SourceProductBaseCode=MS
  Leg : mblibv1/Bodies/Body  LConnTagsString=CG  RConnTagsString=CS1|CS2  UpdateFromCAD=off  DialogClass=MechanicalBodyBlock  Mass=leg_mass  MassUnits=kg  InertiaUnits=kg*m^2  Inertia=zeros(3)  Shape=Cylinder  ShapeDims=[1 1]  ShapeUnits=m  ShapeUse=false  Density=1  DensityUnits=kg/m^3  DensityUse=false  GraphicsMode=CONVHULL  BodyColorSelMode=COLORPALETTE  BodyColor=[0 1 0]  AttachedToCS=CG  CG=Left$CG$[0 0 0]$Adjoining$Adjoining$m$[0 0 0]$Euler X-Y-Z$deg$Adjoining$true$none  WorkingFrames=Right$CS1$[0 0 0]$Adjoining$Adjoining$m$[0 0 0]$Euler X-Y-Z$deg$Adjoining$true$none#Right$CS2$[0 0 0]$Adjoining$Adjoining$m$[0 0 0]$Euler X-Y-Z$deg$Adjoining$true$none  CGPos=[0 0 0]  CGRot=[0 0 0]  CS0Pos=[]  CS0Rot=[]  CS1Pos=[0 0 0]  CS1Rot=[0 0 0]  CS2Pos=[0 0 0]  CS2Rot=[0 0 0]  CS3Pos=[]  CS3Rot=[]  CS4Pos=[]  CS4Rot=[]  CS5Pos=[]  CS5Rot=[]  CS6Pos=[]  CS6Rot=[]  CS7Pos=[]  CS7Rot=[]  CS8Pos=[]  CS8Rot=[]  CS9Pos=[]  CS9Rot=[]  CS10Pos=[]  CS10Rot=[]  CS11Pos=[]  CS11Rot=[]  CS12Pos=[]  CS12Rot=[]  CS13Pos=[]  CS13Rot=[]  CS14Pos=[]  CS14Rot=[]  CS15Pos=[]  CS15Rot=[]  CS16Pos=[]  CS16Rot=[]  CS17Pos=[]  CS17Rot=[]  CS18Pos=[]  CS18Rot=[]  CS19Pos=[]  CS19Rot=[]  CS20Pos=[]  CS20Rot=[]
      settings: SourceProductName=Simscape Multibody  SourceProductBaseCode=MS
  Mechanical Branching Bar : mblibv1/Utilities/Mechanical Branching Bar  LConnTagsString=_newl0  RConnTagsString=SA0|SA1  UpdateFromCAD=off  DialogClass=MechanicalBranchingBarBlock  NumSAPorts=2
      settings: SourceProductName=Simscape Multibody  SourceProductBaseCode=MS
  Prismatic : mblibv1/Joints/Prismatic  LConnTagsString=__newl0|SA1  RConnTagsString=__newr0  UpdateFromCAD=off  NumSAPorts=1  CutJoint=on  MarkAsCut=off  Primitives=prismatic  PrimitiveProps=P1$Follower$p_axis$prismatic  DialogClass=JointBlock  P1Axis=p_axis
      settings: SourceProductName=Simscape Multibody  SourceProductBaseCode=MS
  Vector Concatenate : Concatenate  NumInputs=3
  End effector port : PMIOPort  Port=1  Side=Right
  Sphere port 1 : PMIOPort  Port=2  Side=Left
  Sphere port 2 : PMIOPort  Port=3  Side=Left
  State : Outport
  wires:
  Joint Sensor/1 -> State/1
  Vector Concatenate/1 -> Joint Actuator/1
  Integrator1/1 -> Vector Concatenate/1
  Integrator/1 -> Integrator1/1, Vector Concatenate/2
  Reaction/1 -> Integrator/1, Vector Concatenate/3
  connections:
  End effector port/RConn1 -- Prismatic/RConn1
  In-plane/RConn1 -- Leg/RConn1
  Leg/LConn1 -- Prismatic/LConn1
  In-plane/LConn1 -- Sphere port 1/RConn1
  In-plane1/LConn1 -- Sphere port 2/RConn1
  In-plane1/RConn1 -- Leg/RConn2
  Mechanical Branching Bar/LConn1 -- Prismatic/LConn2
  Joint Actuator/RConn1 -- Mechanical Branching Bar/RConn1
  Joint Sensor/LConn1 -- Mechanical Branching Bar/RConn2

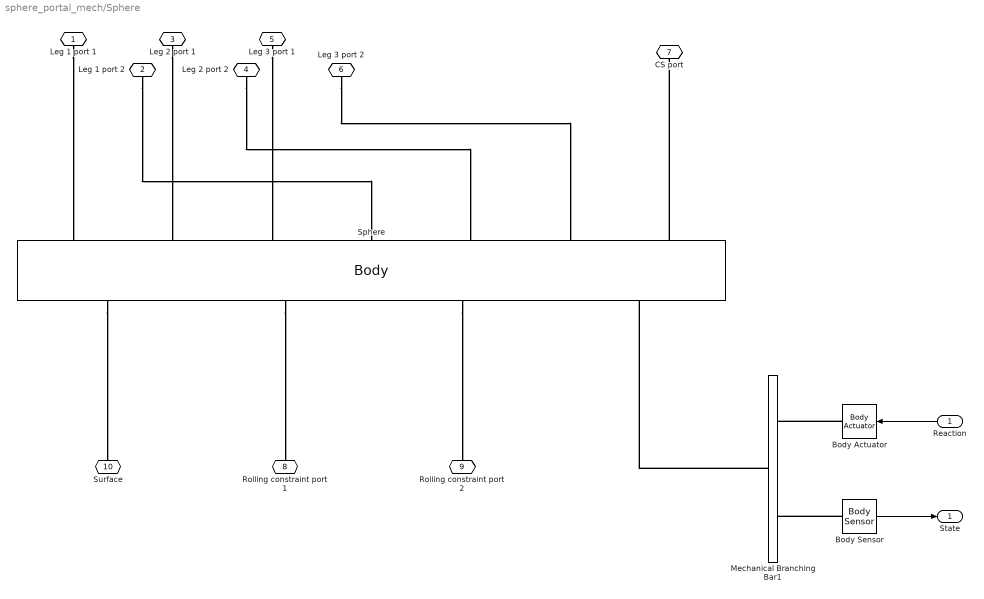
== system sphere_portal_mech/Sphere ==
  Reaction : Inport  OutDataTypeStr=double
  Body Actuator : mblibv1/Sensors &  Actuators/Body Actuator  UpdateFromCAD=off  PhysicalDomain=Mechanical  PortType=blob  ActuationStyle=Force  AngleUnits=deg  ArcVelocityUnits=deg/s  ArcAccelerationUnits=deg/s^2  CoordPositionUnits=m  VelocityUnits=m/s  AccelerationUnits=m/s^2  ForceUnits=N  TorqueUnits=N*m  ActiveIO=on  Width=6  DialogClass=MechanicalActuatorBlock  ReferenceFrame=Absolute (World)  Angle=off  CoordPosition=on  Force=on  Torque=on
      settings: SourceProductName=Simscape Multibody  SourceProductBaseCode=MS
  Body Sensor : mblibv1/Sensors &  Actuators/Body Sensor  UpdateFromCAD=off  PhysicalDomain=Mechanical  PortType=blob  Muxed=on  Pose=on  Angle=on  AngleUnits=deg  ArcVelocity=on  ArcVelocityUnits=rad/s  ArcAcceleration=on  ArcAccelerationUnits=rad/s^2  CoordPosition=on  CoordPositionUnits=m  Velocity=on  VelocityUnits=m/s  Acceleration=on  AccelerationUnits=m/s^2  Quaternion=on  QuaternionDT=off  QuaternionDDT=off  QuaternionUnits=off  OutputVector=[1]  ActiveIO=on  Width=24  DialogClass=MechanicalSensorBlock  ReferenceFrame=Absolute (World)
      settings: SourceProductName=Simscape Multibody  SourceProductBaseCode=MS
  Mechanical Branching Bar1 : mblibv1/Utilities/Mechanical Branching Bar  LConnTagsString=_newl0  RConnTagsString=SA0|SA1  UpdateFromCAD=off  DialogClass=MechanicalBranchingBarBlock  NumSAPorts=2
      settings: SourceProductName=Simscape Multibody  SourceProductBaseCode=MS
  Sphere : mblibv1/Bodies/Body  LConnTagsString=CG|CS8|CS9|CS10  RConnTagsString=CS1|CS2|CS3|CS4|CS5|CS6|CS7  UpdateFromCAD=off  DialogClass=MechanicalBodyBlock  Mass=sphere_mass  MassUnits=kg  InertiaUnits=kg*m^2  Inertia=sphere_inertia_coef*sphere_mass*sphere_radius^2*eye(3)  Shape=Cylinder  ShapeDims=[1 1]  ShapeUnits=m  ShapeUse=false  Density=1  DensityUnits=kg/m^3  DensityUse=false  GraphicsMode=EQELLIPSE  BodyColorSelMode=COLORPALETTE  BodyColor=[0 0 0]  AttachedToCS=CG  CG=Left$CG$[0; 0; 0]$Adjoining$Adjoining$m$[0 0 0]$Euler X-Y-Z$deg$Adjoining$true$none  WorkingFrames=Right$CS1$cube_side_center(:, 1)'$CG$CG$m$[0 0 0]$Euler X-Y-Z$deg$CG$true$none#Right$CS2$cube_side_center(:, 2)'$CG$CG$m$[0 0 0]$Euler X-Y-Z$deg$CG$true$none#Right$CS3$cube_side_center(:, 3)'$CG$CG$m$[0 0 0]$Euler X-Y-Z$deg$CG$true$none#Right$CS4$cube_side_center(:, 4)'$CG$CG$m$[0 0 0]$Euler X-Y-Z$deg$CG$true$none#Right$CS5$cube_side_center(:, 5)'$CG$CG$m$[0 0 0]$Euler X-Y-Z$deg$CG$true$none#Right$CS6$cube_side_center(:, 6)'$CG$CG$m$[0 0 0]$Euler X-Y-Z$deg$CG$true$none#Right$CS7$[0; 0; 0]$CG$CG$m$[0 0 0]$Euler X-Y-Z$deg$CG$true$none#Left$CS8$[0; 0; 0]$CG$CG$m$[0 0 0]$Euler X-Y-Z$deg$CG$true$none#Left$CS9$[0; 0; 0]$CG$CG$m$[0 0 0]$Euler X-Y-Z$deg$CG$true$none#Left$CS10$[0; 0; 0]$CG$CG$m$[0 0 0]$Euler X-Y-Z$deg$CG$true$none  CGPos=[0; 0; 0]  CGRot=[0 0 0]  CS0Pos=[]  CS0Rot=[]  CS1Pos=cube_side_center(:, 1)'  CS1Rot=[0 0 0]  CS2Pos=cube_side_center(:, 2)'  CS2Rot=[0 0 0]  CS3Pos=cube_side_center(:, 3)'  CS3Rot=[0 0 0]  CS4Pos=cube_side_center(:, 4)'  CS4Rot=[0 0 0]  CS5Pos=cube_side_center(:, 5)'  CS5Rot=[0 0 0]  CS6Pos=cube_side_center(:, 6)'  CS6Rot=[0 0 0]  CS7Pos=[0; 0; 0]  CS7Rot=[0 0 0]  CS8Pos=[0; 0; 0]  CS8Rot=[0 0 0]  CS9Pos=[0; 0; 0]  CS9Rot=[0 0 0]  CS10Pos=[0; 0; 0]  CS10Rot=[0 0 0]  CS11Pos=[]  CS11Rot=[]  CS12Pos=[]  CS12Rot=[]  CS13Pos=[]  CS13Rot=[]  CS14Pos=[]  CS14Rot=[]  CS15Pos=[]  CS15Rot=[]  CS16Pos=[]  CS16Rot=[]  CS17Pos=[]  CS17Rot=[]  CS18Pos=[]  CS18Rot=[]  CS19Pos=[]  CS19Rot=[]  CS20Pos=[]  CS20Rot=[]
      settings: SourceProductName=Simscape Multibody  SourceProductBaseCode=MS
  Leg 1 port 1 : PMIOPort  Port=1  Side=Right
  Leg 1 port 2 : PMIOPort  Port=2  Side=Right
  Leg 2 port 1 : PMIOPort  Port=3  Side=Right
  Leg 2 port 2 : PMIOPort  Port=4  Side=Right
  Leg 3 port 1 : PMIOPort  Port=5  Side=Right
  Leg 3 port 2 : PMIOPort  Port=6  Side=Right
  CS port : PMIOPort  Port=7  Side=Right
  Rolling constraint port 1 : PMIOPort  Port=8  Side=Left
  Rolling constraint port 2 : PMIOPort  Port=9  Side=Left
  Surface : PMIOPort  Port=10  Side=Left
  State : Outport  OutDataTypeStr=double
  wires:
  Reaction/1 -> Body Actuator/1
  Body Sensor/1 -> State/1
  connections:
  Sphere/LConn3 -- Rolling constraint port 2/RConn1
  Sphere/LConn2 -- Rolling constraint port 1/RConn1
  Sphere/LConn1 -- Surface/RConn1
  Sphere/RConn7 -- CS port/RConn1
  Leg 2 port 2/RConn1 -- Sphere/RConn5
  Leg 3 port 2/RConn1 -- Sphere/RConn6
  Leg 1 port 2/RConn1 -- Sphere/RConn4
  Leg 2 port 1/RConn1 -- Sphere/RConn2
  Leg 3 port 1/RConn1 -- Sphere/RConn3
  Leg 1 port 1/RConn1 -- Sphere/RConn1
  Mechanical Branching Bar1/LConn1 -- Sphere/LConn4
  Body Sensor/LConn1 -- Mechanical Branching Bar1/RConn2
  Body Actuator/RConn1 -- Mechanical Branching Bar1/RConn1

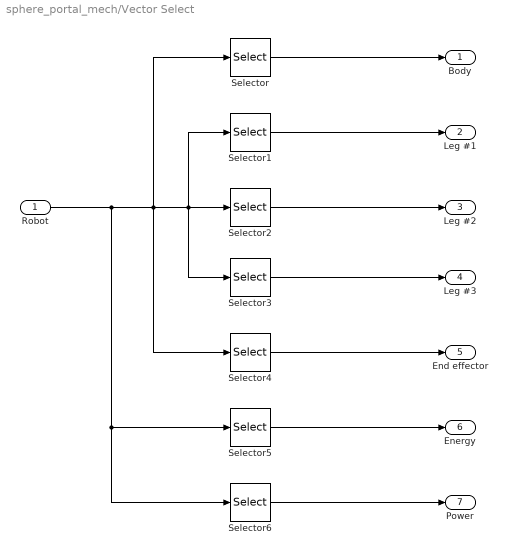
== system sphere_portal_mech/Vector Select ==
  Robot : Inport
  Selector : Selector  IndexOptions=Starting index (dialog)  Indices=1  OutputSizes=6
  Selector1 : Selector  IndexOptions=Starting index (dialog)  Indices=7  OutputSizes=1
  Selector2 : Selector  IndexOptions=Starting index (dialog)  Indices=8  OutputSizes=1
  Selector3 : Selector  IndexOptions=Starting index (dialog)  Indices=9  OutputSizes=1
  Selector4 : Selector  IndexOptions=Starting index (dialog)  Indices=10  OutputSizes=6
  Selector5 : Selector  IndexOptions=Starting index (dialog)  Indices=16  OutputSizes=1
  Selector6 : Selector  IndexOptions=Starting index (dialog)  Indices=17  OutputSizes=1
  Body : Outport
  Leg #1 : Outport  Port=2
  Leg #2 : Outport  Port=3
  Leg #3 : Outport  Port=4
  End effector : Outport  Port=5
  Energy : Outport  Port=6
  Power : Outport  Port=7
  wires:
  Selector4/1 -> End effector/1
  Selector2/1 -> Leg #2/1
  Selector1/1 -> Leg #1/1
  Selector3/1 -> Leg #3/1
  Selector/1 -> Body/1
  Robot/1 -> Selector5/1, Selector6/1, Selector4/1, Selector/1, Selector3/1, Selector1/1, Selector2/1
  Selector5/1 -> Energy/1
  Selector6/1 -> Power/1

== system sphere_portal_mech/Environment/Plane ==
  Constraint Point : mblibv1/Bodies/Body  LConnTagsString=CG  RConnTagsString=CS5  UpdateFromCAD=off  DialogClass=MechanicalBodyBlock  Mass=0  MassUnits=kg  InertiaUnits=kg*m^2  Inertia=zeros(3)  Shape=Cylinder  ShapeDims=[1 1]  ShapeUnits=m  ShapeUse=false  Density=1  DensityUnits=kg/m^3  DensityUse=false  GraphicsMode=CONVHULL  BodyColorSelMode=COLORPALETTE  BodyColor=[0.23137 0.44314 0.33725]  AttachedToCS=CG  CG=Left$CG$[0 0 0]$WORLD$WORLD$m$[0 0 0]$Euler X-Y-Z$deg$WORLD$true$none  WorkingFrames=Right$CS5$[0 0 0]$Adjoining$Adjoining$m$[0 0 0]$Euler X-Y-Z$deg$WORLD$true$none  CGPos=[0 0 0]  CGRot=[0 0 0]  CS0Pos=[]  CS0Rot=[]  CS1Pos=[]  CS1Rot=[]  CS2Pos=[]  CS2Rot=[]  CS3Pos=[]  CS3Rot=[]  CS4Pos=[]  CS4Rot=[]  CS5Pos=[0 0 0]  CS5Rot=[0 0 0]  CS6Pos=[]  CS6Rot=[]  CS7Pos=[]  CS7Rot=[]  CS8Pos=[]  CS8Rot=[]  CS9Pos=[]  CS9Rot=[]  CS10Pos=[]  CS10Rot=[]  CS11Pos=[]  CS11Rot=[]  CS12Pos=[]  CS12Rot=[]  CS13Pos=[]  CS13Rot=[]  CS14Pos=[]  CS14Rot=[]  CS15Pos=[]  CS15Rot=[]  CS16Pos=[]  CS16Rot=[]  CS17Pos=[]  CS17Rot=[]  CS18Pos=[]  CS18Rot=[]  CS19Pos=[]  CS19Rot=[]  CS20Pos=[]  CS20Rot=[]
      settings: SourceProductName=Simscape Multibody  SourceProductBaseCode=MS
  Ground : mblibv1/Bodies/Ground  UpdateFromCAD=off  LeftPortType=env  RightPortType=workingframe  PhysicalDomain=Mechanical  DialogClass=GroundBlock  CoordPosition=[0 0 -sphere_radius]  CoordPositionUnits=m  StateVectorMgrId=0  MachineId=[1 0]  ShowEnvPort=on  ParameterChecksum=[2331306565, 3420490137, 3105387195, 2316833504]  TopologyChecksum=[2312807192, 2535003239, 2113725408, 404379218]
      settings: SourceProductName=Simscape Multibody  SourceProductBaseCode=MS
  Machine Environment : mblibv1/Bodies/Machine Environment  Tag=Factory ground  PortType=env  PhysicalDomain=Mechanical  DialogTemplateClass=MECH.MachineEnvironment  SyncWhenCopied=off  Gravity=[0 0 -9.81]  GravityUnits=m/s^2  GravityAsSignal=off  Dimensionality=3D Only  AnalysisType=Forward dynamics  LinearAssemblyTolerance=1e-3  LinearAssemblyToleranceUnits=m  AngularAssemblyTolerance=1e-3  AngularAssemblyToleranceUnits=rad  ConstraintSolverType=Stabilizing  ConstraintRelTolerance=1e-4  ConstraintAbsTolerance=1e-4  UseRobustSingularityHandling=off  RedundancyAnalysisToleranceType=Automatically select tolerance  RedundancyAnalysisTolerance=1e-14  StatePerturbationType=Fixed  PerturbationSize=1e-5  VisualizeMachine=on  BodyVisualizationType=Use model default body geometries  BodyColorSelMode=Use model default  DefaultBodyColor=[1 0 0]
      settings: SourceProductName=Simscape Multibody  SourceProductBaseCode=MS
  Plane : mblibv1/Bodies/Body  LConnTagsString=CG  RConnTagsString=CS1  UpdateFromCAD=off  DialogClass=MechanicalBodyBlock  Mass=1  MassUnits=kg  InertiaUnits=kg*m^2  Inertia=(1/12)*[400 0 0;0 400 0;0 0 800]  Shape=Cylinder  ShapeDims=[1 1]  ShapeUnits=m  ShapeUse=false  Density=1  DensityUnits=kg/m^3  DensityUse=false  GraphicsMode=CONVHULL  BodyColorSelMode=COLORPALETTE  BodyColor=[0.23137 0.44314 0.33725]  AttachedToCS=CG  CG=Left$CG$[0 0 0]$CS1$CS1$m$[0 0 0]$Euler X-Y-Z$deg$WORLD$true$none  WorkingFrames=Right$CS1$[0 0 0]$Adjoining$Adjoining$m$[0 0 0]$Euler X-Y-Z$deg$WORLD$true$none#Right$CS2$[width width 0]$CG$CG$m$[0 0 0]$Euler X-Y-Z$deg$WORLD$false$none#Right$CS3$[width -width 0]$CG$CG$m$[0 0 0]$Euler X-Y-Z$deg$WORLD$false$none#Right$CS4$[-width width 0]$CG$CG$m$[0 0 0]$Euler X-Y-Z$deg$WORLD$false$none#Right$CS5$[-width -width 0]$CG$CG$m$[0 0 0]$Euler X-Y-Z$deg$WORLD$false$none  CGPos=[0 0 0]  CGRot=[0 0 0]  CS0Pos=[]  CS0Rot=[]  CS1Pos=[0 0 0]  CS1Rot=[0 0 0]  CS2Pos=[width width 0]  CS2Rot=[0 0 0]  CS3Pos=[width -width 0]  CS3Rot=[0 0 0]  CS4Pos=[-width width 0]  CS4Rot=[0 0 0]  CS5Pos=[-width -width 0]  CS5Rot=[0 0 0]  CS6Pos=[]  CS6Rot=[]  CS7Pos=[]  CS7Rot=[]  CS8Pos=[]  CS8Rot=[]  CS9Pos=[]  CS9Rot=[]  CS10Pos=[]  CS10Rot=[]  CS11Pos=[]  CS11Rot=[]  CS12Pos=[]  CS12Rot=[]  CS13Pos=[]  CS13Rot=[]  CS14Pos=[]  CS14Rot=[]  CS15Pos=[]  CS15Rot=[]  CS16Pos=[]  CS16Rot=[]  CS17Pos=[]  CS17Rot=[]  CS18Pos=[]  CS18Rot=[]  CS19Pos=[]  CS19Rot=[]  CS20Pos=[]  CS20Rot=[]
      settings: SourceProductName=Simscape Multibody  SourceProductBaseCode=MS
  Weld : mblibv1/Joints/Weld  LConnTagsString=__newl0  RConnTagsString=__newr0  UpdateFromCAD=off  NumSAPorts=0  CutJoint=off  MarkAsCut=off  Primitives=weld  PrimitiveProps=W$WORLD$[0 0 0]$weld  DialogClass=JointBlock  WAxis=[0 0 0]
      settings: SourceProductName=Simscape Multibody  SourceProductBaseCode=MS
  Weld1 : mblibv1/Joints/Weld  LConnTagsString=__newl0  RConnTagsString=__newr0  UpdateFromCAD=off  NumSAPorts=0  CutJoint=off  MarkAsCut=off  Primitives=weld  PrimitiveProps=W$WORLD$[0 0 0]$weld  DialogClass=JointBlock  WAxis=[0 0 0]
      settings: SourceProductName=Simscape Multibody  SourceProductBaseCode=MS
  Point : PMIOPort  Port=1  Side=Left
  connections:
  Weld1/RConn1 -- Constraint Point/RConn1
  Machine Environment/RConn1 -- Ground/LConn1
  Ground/RConn1 -- Weld/LConn1
  Plane/LConn1 -- Weld1/LConn1
  Plane/RConn1 -- Weld/RConn1
  Point/RConn1 -- Constraint Point/LConn1

== system sphere_portal_mech/Environment/Rolling constraint ==
  note: vel_x = + omega_y
      | vel_y = - omega_x
  First rolling constraint : mblibv1/Constraints &  Drivers/Velocity Driver  LConnTagsString=__newl0  RConnTagsString=__newr0  UpdateFromCAD=off  DialogClass=ConstantVelocityConstraint  NumSAPorts=0  Unit_V=m/s  Unit_Omega=rad/s  Coef_V_Base=[1 0 0]  Csys_V_Base=World  Coef_Omega_Base=[0 -1 0]  Csys_Omega_Base=World  Coef_V_Follower=[0 0 0]  Csys_V_Follower=World  Coef_Omega_Follower=[0 0 0]  Csys_Omega_Follower=World
      settings: SourceProductName=Simscape Multibody  SourceProductBaseCode=MS
  Ground1 : mblibv1/Bodies/Ground  UpdateFromCAD=off  LeftPortType=env  RightPortType=workingframe  PhysicalDomain=Mechanical  DialogClass=GroundBlock  CoordPosition=[0 0 0]  CoordPositionUnits=m  StateVectorMgrId=-1  MachineId=[0 0]  ShowEnvPort=off  ParameterChecksum=[0 0 0 0]  TopologyChecksum=[0 0 0 0]
      settings: SourceProductName=Simscape Multibody  SourceProductBaseCode=MS
  Ground2 : mblibv1/Bodies/Ground  UpdateFromCAD=off  LeftPortType=env  RightPortType=workingframe  PhysicalDomain=Mechanical  DialogClass=GroundBlock  CoordPosition=[0 0 0]  CoordPositionUnits=m  StateVectorMgrId=-1  MachineId=[0 0]  ShowEnvPort=off  ParameterChecksum=[0 0 0 0]  TopologyChecksum=[0 0 0 0]
      settings: SourceProductName=Simscape Multibody  SourceProductBaseCode=MS
  Second rolling constraint : mblibv1/Constraints &  Drivers/Velocity Driver  LConnTagsString=__newl0  RConnTagsString=__newr0  UpdateFromCAD=off  DialogClass=ConstantVelocityConstraint  NumSAPorts=0  Unit_V=m/s  Unit_Omega=rad/s  Coef_V_Base=[0 1 0]  Csys_V_Base=World  Coef_Omega_Base=[1 0 0]  Csys_Omega_Base=World  Coef_V_Follower=[0 0 0]  Csys_V_Follower=World  Coef_Omega_Follower=[0 0 0]  Csys_Omega_Follower=World
      settings: SourceProductName=Simscape Multibody  SourceProductBaseCode=MS
  Constraint 1 : PMIOPort  Port=1  Side=Left
  Constraint 2 : PMIOPort  Port=2  Side=Left
  connections:
  First rolling constraint/RConn1 -- Ground1/RConn1
  Second rolling constraint/RConn1 -- Ground2/RConn1
  Constraint 2/RConn1 -- Second rolling constraint/LConn1
  Constraint 1/RConn1 -- First rolling constraint/LConn1
